simulink model "simulations"  (R2023b)
settings: Solver=VariableStepAuto  StartTime=0.0  StopTime=56  RelTol=1e-3
values from neighbouring files (symbols this model uses):
  F = pinv((Cd*(eye(4) - (Ad+Bd*K))^(-1)*Bd))    [pendulum_control.m]
  H = -KH(end)    [pendulum_control.m]
  K = - place(Ad, Bd, pK)    [pendulum_control.m]
  K_int = KH(1:end-1)    [pendulum_control.m]
  T = 0.01    [pendulum_control.m]
undefined symbols (not defined in the file or in its folder): DiscIntNeverNeededParam
libraries: cstblocks x10, eeLuenbergerObserver x5
settings Model: Creator=matia  LastModifiedBy=matia
settings SolverCC: MaxConsecutiveMinStep=3

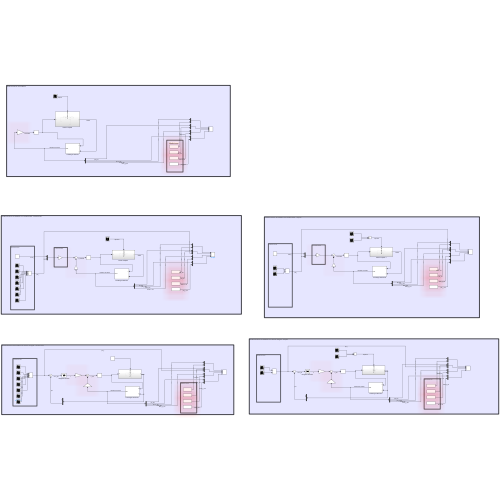
[thumbnail: Simulink's stored preview of the top-level diagram]
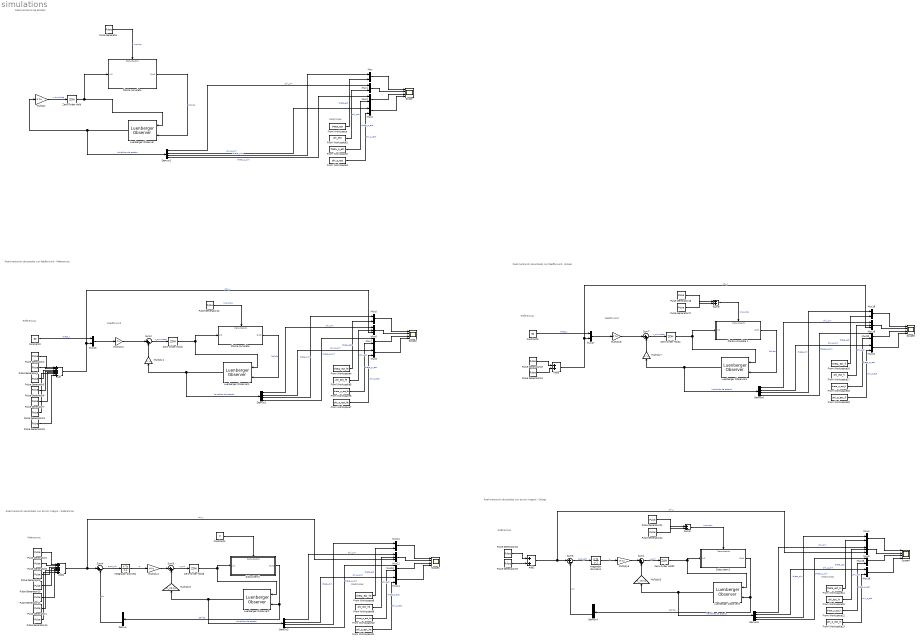
== system simulations ==
  note: Realimentación de estados con acción integral - Golpes
  note: Realimentación de estados con acción integral - Referencias
  note: Realimentación de estados con feedforward - Golpes
  note: Realimentación de estados con feedforward - Referencias
  note: Realimentación de estados
  note: Mediciones
  note: Referencias
  note: Referencias
  note: Feedforward
  note: Mediciones
  note: Referencias
  note: Mediciones
  note: Referencias
  note: Feedforward
  Add : Sum  Inputs=+++++++
  Add1 : Sum  Inputs=+++++++
  Add2 : Sum
  Add3 : Sum
  Constant1 : Constant  Value=0
  Constant2 : Constant  Value=60
  Constant3 : Constant  Value=60
  Demux : Demux  Outputs=2
  Demux{1..3,5..6} (5 alike) : Demux
  Demux4 : Demux  Outputs=2
  From Workspace : FromWorkspace  VariableName=theta_est  OutDataTypeStr=double  SampleTime=T  OutputAfterFinalValue=Setting to zero
  From Workspace1 : FromWorkspace  VariableName=phi_est  OutDataTypeStr=double  SampleTime=T  OutputAfterFinalValue=Setting to zero
  From Workspace10 : FromWorkspace  VariableName=theta_p_est_he  OutDataTypeStr=double  SampleTime=T
  From Workspace11 : FromWorkspace  VariableName=phi_p_est_he  OutDataTypeStr=double  SampleTime=T
  From Workspace12 : FromWorkspace  VariableName=theta_p_est_hi  OutDataTypeStr=double  SampleTime=T
  From Workspace13 : FromWorkspace  VariableName=phi_p_est_hi  OutDataTypeStr=double  SampleTime=T
  From Workspace14 : FromWorkspace  VariableName=theta_est_hi  OutDataTypeStr=double  SampleTime=T  OutputAfterFinalValue=Setting to zero
  From Workspace15 : FromWorkspace  VariableName=phi_est_hi  OutDataTypeStr=double  SampleTime=T
  From Workspace16 : FromWorkspace  VariableName=theta_est_fi  OutDataTypeStr=double  SampleTime=T  OutputAfterFinalValue=Setting to zero
  From Workspace17 : FromWorkspace  VariableName=phi_est_fi  SampleTime=T  OutputAfterFinalValue=Setting to zero
  From Workspace18 : FromWorkspace  VariableName=theta_p_est_fi  OutDataTypeStr=double  SampleTime=T  OutputAfterFinalValue=Setting to zero
  From Workspace19 : FromWorkspace  VariableName=phi_p_est_fi  OutDataTypeStr=double  SampleTime=T  OutputAfterFinalValue=Setting to zero
  From Workspace2 : FromWorkspace  VariableName=theta_p_est  OutDataTypeStr=double  SampleTime=T  OutputAfterFinalValue=Setting to zero
  From Workspace3 : FromWorkspace  VariableName=phi_p_est  OutDataTypeStr=double  SampleTime=T  OutputAfterFinalValue=Setting to zero
  From Workspace4 : FromWorkspace  VariableName=theta_est_fe  OutDataTypeStr=double  SampleTime=T  OutputAfterFinalValue=Setting to zero
  From Workspace5 : FromWorkspace  VariableName=phi_est_fe  OutDataTypeStr=double  SampleTime=T
  From Workspace6 : FromWorkspace  VariableName=theta_p_est_fe  OutDataTypeStr=double  SampleTime=T
  From Workspace7 : FromWorkspace  VariableName=phi_p_est_fe  OutDataTypeStr=double  SampleTime=T
  From Workspace8 : FromWorkspace  VariableName=theta_est_he  OutDataTypeStr=double  SampleTime=T  OutputAfterFinalValue=Setting to zero
  From Workspace9 : FromWorkspace  VariableName=phi_est_he  OutDataTypeStr=double  SampleTime=T
  Integrador discreto : DiscreteIntegrator  gainval=1/T  SampleTime=T  ICPrevOutput=DiscIntNeverNeededParam  ICPrevScaledInput=DiscIntNeverNeededParam
  Integrador discreto1 : DiscreteIntegrator  gainval=1/T  SampleTime=T  ICPrevOutput=DiscIntNeverNeededParam  ICPrevScaledInput=DiscIntNeverNeededParam
  Luenberger Observer{,1..4} (5 alike) : eeLuenbergerObserver/Luenberger Observer  StateSpaceType=Discrete-time  Ad=Ad  Bd=Bd  Cd=Cd  Dd=Dd  A=1  B=1  C=1  D=1  ObserverDesign=Desired eigenvalues  Ld=1  DesiredEigenvalues=pL  x0=[0;0;0;0]  Tsd=0.1  Ts=T
      settings: LibrarySourceBlock=ee_sl_lib/Observers/Luenberger Observer
  Multiply : Gain  Gain=K  Multiplication=Matrix(K*u)
  Multiply1 : Gain  Gain=K  Multiplication=Matrix(K*u)
  Multiply2 : Gain  Gain=F  Multiplication=Matrix(K*u)
  Multiply3 : Gain  Gain=K_int  Multiplication=Matrix(K*u)
  Multiply4 : Gain  Gain=H  Multiplication=Matrix(K*u)
  Multiply5 : Gain  Gain=K_int  Multiplication=Matrix(K*u)
  Multiply6 : Gain  Gain=H  Multiplication=Matrix(K*u)
  Multiply7 : Gain  Gain=K  Multiplication=Matrix(K*u)
  Multiply8 : Gain  Gain=F  Multiplication=Matrix(K*u)
  Mux{,1..5,7..8,10..11,13..18,20..21} (18 alike) : Mux  Inputs=2
  Mux{6,9,12,19} (4 alike) : Mux  Inputs=3
  Planta completa : Subsystem
      settings: PortSchema="{\"entries\":[{\"content\":{\"sides\":[{\"content\":{\"connectorIds\":[\"In1\"]},\"type\":\"ConnectorPlacement.EquallySpacedRectSide\",\"uuid\":\"327bad0f-c414-403a-b9df-5d815b8b637d\"},{\"content\":{\"connectorIds\":[\"Out1\"],\"side\":\"RIGHT\"},\"type\":\"ConnectorPlacement.EquallySpacedRectSide\",\"uuid\":\"9527d032-ecf2-4fa1-93b0-9f68fe8f2eae\"},{\"content\":{\"connectorIds\":[\"In2\"],\"side\":\"TOP\"},\"type\":\"ConnectorPlacement.EquallySpacedRectSide\",\"uuid\":\"a3d79d93-56b9-460d-b273-a140d39cea96\"}]},\"type\":\"ConnectorPlacement.EquallySpacedConnector\",\"uuid\":\"02353cda-d734-4829-adbd-41d8cd1e3a5e\"}],\"packageUris\":[\"http://schema.mathworks.com/mf0/Connector/R2020b\"],\"version\":\"1.0\"}"
  "Planta completa " : Subsystem
      settings: PortSchema="{\"entries\":[{\"content\":{\"sides\":[{\"content\":{\"connectorIds\":[\"In1\"]},\"type\":\"ConnectorPlacement.EquallySpacedRectSide\",\"uuid\":\"327bad0f-c414-403a-b9df-5d815b8b637d\"},{\"content\":{\"connectorIds\":[\"Out1\"],\"side\":\"RIGHT\"},\"type\":\"ConnectorPlacement.EquallySpacedRectSide\",\"uuid\":\"9527d032-ecf2-4fa1-93b0-9f68fe8f2eae\"},{\"content\":{\"connectorIds\":[\"In2\"],\"side\":\"TOP\"},\"type\":\"ConnectorPlacement.EquallySpacedRectSide\",\"uuid\":\"a3d79d93-56b9-460d-b273-a140d39cea96\"}]},\"type\":\"ConnectorPlacement.EquallySpacedConnector\",\"uuid\":\"02353cda-d734-4829-adbd-41d8cd1e3a5e\"}],\"packageUris\":[\"http://schema.mathworks.com/mf0/Connector/R2020b\"],\"version\":\"1.0\"}"
  Planta completa 1 : Subsystem
      settings: PortSchema="{\"entries\":[{\"content\":{\"sides\":[{\"content\":{\"connectorIds\":[\"In1\"]},\"type\":\"ConnectorPlacement.EquallySpacedRectSide\",\"uuid\":\"327bad0f-c414-403a-b9df-5d815b8b637d\"},{\"content\":{\"connectorIds\":[\"Out1\"],\"side\":\"RIGHT\"},\"type\":\"ConnectorPlacement.EquallySpacedRectSide\",\"uuid\":\"9527d032-ecf2-4fa1-93b0-9f68fe8f2eae\"},{\"content\":{\"connectorIds\":[\"In2\"],\"side\":\"TOP\"},\"type\":\"ConnectorPlacement.EquallySpacedRectSide\",\"uuid\":\"a3d79d93-56b9-460d-b273-a140d39cea96\"}]},\"type\":\"ConnectorPlacement.EquallySpacedConnector\",\"uuid\":\"02353cda-d734-4829-adbd-41d8cd1e3a5e\"}],\"packageUris\":[\"http://schema.mathworks.com/mf0/Connector/R2020b\"],\"version\":\"1.0\"}"
  Pulse Generator : DiscretePulseGenerator  PulseType=Time based  Amplitude=-8000  Period=100  PulseWidth=0.1  PhaseDelay=0.4
  Pulse Generator1 : DiscretePulseGenerator  PulseType=Time based  Amplitude=0  Period=100  PulseWidth=8  PhaseDelay=40
  Pulse Generator10 : DiscretePulseGenerator  PulseType=Time based  Amplitude=45  Period=100  PulseWidth=8  PhaseDelay=24
  Pulse Generator11 : DiscretePulseGenerator  PulseType=Time based  Amplitude=10  Period=100  PulseWidth=8  PhaseDelay=32
  Pulse Generator12 : DiscretePulseGenerator  PulseType=Time based  Amplitude=-8000  Period=100  PulseWidth=0.1  PhaseDelay=100
  Pulse Generator13 : DiscretePulseGenerator  PulseType=Time based  Amplitude=-30  Period=100  PulseWidth=8  PhaseDelay=40-0.445
  Pulse Generator14 : DiscretePulseGenerator  PulseType=Time based  Amplitude=20  Period=100  PulseWidth=8  PhaseDelay=48
  Pulse Generator15 : DiscretePulseGenerator  PulseType=Time based  Amplitude=-10  Period=100  PulseWidth=8  PhaseDelay=48-0.445
  Pulse Generator16 : DiscretePulseGenerator  PulseType=Time based  Amplitude=50000  Period=100  PulseWidth=0.01  PhaseDelay=4.77
  Pulse Generator17 : DiscretePulseGenerator  PulseType=Time based  Amplitude=-80000  Period=100  PulseWidth=0.01  PhaseDelay=25.8
  Pulse Generator18 : DiscretePulseGenerator  PulseType=Time based  Amplitude=45  Period=100  PulseWidth=20
  Pulse Generator19 : DiscretePulseGenerator  PulseType=Time based  Amplitude=-10  Period=100  PulseWidth=90  PhaseDelay=20
  Pulse Generator2 : DiscretePulseGenerator  PulseType=Time based  Amplitude=30  Period=100  PulseWidth=8
  Pulse Generator21 : DiscretePulseGenerator  PulseType=Time based  Amplitude=80000  Period=100  PulseWidth=0.01  PhaseDelay=8.136
  Pulse Generator22 : DiscretePulseGenerator  PulseType=Time based  Amplitude=80000  Period=100  PulseWidth=0.01  PhaseDelay=34.135
  Pulse Generator23 : DiscretePulseGenerator  PulseType=Time based  Amplitude=30  Period=100  PulseWidth=20
  Pulse Generator24 : DiscretePulseGenerator  PulseType=Time based  Amplitude=20  Period=100  PulseWidth=90  PhaseDelay=20
  Pulse Generator3 : DiscretePulseGenerator  PulseType=Time based  Amplitude=-20  Period=100  PulseWidth=8
  Pulse Generator4 : DiscretePulseGenerator  PulseType=Time based  Amplitude=-30  Period=100  PulseWidth=8  PhaseDelay=8-0.445
  Pulse Generator5 : DiscretePulseGenerator  PulseType=Time based  Amplitude=-10  Period=100  PulseWidth=8  PhaseDelay=16-0.445
  Pulse Generator6 : DiscretePulseGenerator  PulseType=Time based  Amplitude=20  Period=100  PulseWidth=8  PhaseDelay=24-0.445
  Pulse Generator7 : DiscretePulseGenerator  PulseType=Time based  Amplitude=0  Period=100  PulseWidth=8  PhaseDelay=32-0.445
  Pulse Generator8 : DiscretePulseGenerator  PulseType=Time based  Amplitude=0  Period=100  PulseWidth=8  PhaseDelay=8
  Pulse Generator9 : DiscretePulseGenerator  PulseType=Time based  Amplitude=20  Period=100  PulseWidth=8  PhaseDelay=16
  Scope{,2..5} (5 alike) : Scope  NumInputPorts=4
  Subsystem1 : Subsystem
      settings: PortSchema="{\"entries\":[{\"content\":{\"sides\":[{\"content\":{\"connectorIds\":[\"In1\"]},\"type\":\"ConnectorPlacement.EquallySpacedRectSide\",\"uuid\":\"327bad0f-c414-403a-b9df-5d815b8b637d\"},{\"content\":{\"connectorIds\":[\"Out1\"],\"side\":\"RIGHT\"},\"type\":\"ConnectorPlacement.EquallySpacedRectSide\",\"uuid\":\"9527d032-ecf2-4fa1-93b0-9f68fe8f2eae\"},{\"content\":{\"connectorIds\":[\"In2\"],\"side\":\"TOP\"},\"type\":\"ConnectorPlacement.EquallySpacedRectSide\",\"uuid\":\"a3d79d93-56b9-460d-b273-a140d39cea96\"}]},\"type\":\"ConnectorPlacement.EquallySpacedConnector\",\"uuid\":\"02353cda-d734-4829-adbd-41d8cd1e3a5e\"}],\"packageUris\":[\"http://schema.mathworks.com/mf0/Connector/R2020b\"],\"version\":\"1.0\"}"
  Subsystem2 : Subsystem
      settings: PortSchema="{\"entries\":[{\"content\":{\"sides\":[{\"content\":{\"connectorIds\":[\"In1\"]},\"type\":\"ConnectorPlacement.EquallySpacedRectSide\",\"uuid\":\"327bad0f-c414-403a-b9df-5d815b8b637d\"},{\"content\":{\"connectorIds\":[\"Out1\"],\"side\":\"RIGHT\"},\"type\":\"ConnectorPlacement.EquallySpacedRectSide\",\"uuid\":\"9527d032-ecf2-4fa1-93b0-9f68fe8f2eae\"},{\"content\":{\"connectorIds\":[\"In2\"],\"side\":\"TOP\"},\"type\":\"ConnectorPlacement.EquallySpacedRectSide\",\"uuid\":\"a3d79d93-56b9-460d-b273-a140d39cea96\"}]},\"type\":\"ConnectorPlacement.EquallySpacedConnector\",\"uuid\":\"02353cda-d734-4829-adbd-41d8cd1e3a5e\"}],\"packageUris\":[\"http://schema.mathworks.com/mf0/Connector/R2020b\"],\"version\":\"1.0\"}"
  Sum{1..3,6..8} (6 alike) : Sum  Inputs=|++
  Sum4 : Sum  Inputs=|+-
  Sum5 : Sum  Inputs=|+-
  Zero-Order Hold{,1..4} (5 alike) : ZeroOrderHold  SampleTime=T
  wires:
  Demux1/1 -> Mux1/1  "phi_sim"
  Demux1/3 -> Mux/1  "theta_sim"
  From Workspace/1 -> Mux/2  "theta_est"
  From Workspace1/1 -> Mux1/2  "phi_est"
  From Workspace2/1 -> Mux2/2  "theta_p_est"
  From Workspace3/1 -> Mux3/2  "phi_p_est"
  Demux1/2 -> Mux3/1  "phi_p_sim"
  Demux1/4 -> Mux2/1  "theta_p_sim"
  Mux/1 -> Scope/1
  Mux1/1 -> Scope/2
  Mux2/1 -> Scope/3
  Mux3/1 -> Scope/4
  Luenberger Observer/1 -> Multiply/1, Demux1/1  "Variables de estado"
  Demux2/3 -> Mux5/1  "theta_sim"
  Mux8/1 -> Scope2/4
  Mux5/1 -> Scope2/1
  Mux7/1 -> Scope2/3
  Mux6/1 -> Scope2/2
  Luenberger Observer1/1 -> Multiply1/1, Demux2/1  "Variables de estado"
  Demux2/1 -> Mux6/1  "phi_sim"
  Demux2/2 -> Mux8/1  "phi_p_sim"
  From Workspace6/1 -> Mux7/2  "theta_p_est"
  Demux2/4 -> Mux7/1  "theta_p_sim"
  From Workspace7/1 -> Mux8/2  "phi_p_est"
  From Workspace4/1 -> Mux5/2  "theta_est"
  "Planta completa "/1(Out1) -> Luenberger Observer1/2  "Salida"
  Multiply1/1 -> Sum2/2
  Sum2/1 -> Zero-Order Hold1/1  "u_simulada"
  Mux10/1 -> Multiply2/1
  Constant2/1 -> Mux10/1  "theta_r"
  Pulse Generator2/1 -> Add/1
  Pulse Generator4/1 -> Add/2
  Pulse Generator5/1 -> Add/3
  Pulse Generator6/1 -> Add/4
  Pulse Generator7/1 -> Add/5
  Add/1 -> Mux6/3, Mux10/2  "phi_r"
  Multiply2/1 -> Sum2/1
  Multiply4/1 -> Sum3/1
  Multiply3/1 -> Sum3/2
  Demux3/2 -> Mux14/1  "phi_p_sim"
  Luenberger Observer2/1 -> Multiply3/1, Demux3/1  "Variables de estado"
  From Workspace8/1 -> Mux11/2  "theta_est"
  Mux12/1 -> Scope3/2
  Mux13/1 -> Scope3/3
  Demux3/3 -> Mux11/1  "theta_sim"
  Subsystem2/1(Out1) -> Demux/1, Luenberger Observer2/2  "Salida"
  Mux14/1 -> Scope3/4
  Sum3/1 -> Zero-Order Hold3/1  "u_sim"
  From Workspace10/1 -> Mux13/2  "theta_p_est"
  Demux3/4 -> Mux13/1  "theta_p_sim"
  Mux11/1 -> Scope3/1
  Demux3/1 -> Mux12/1  "phi_sim"
  From Workspace11/1 -> Mux14/2  "phi_p_est"
  Sum4/1 -> Integrador discreto/1  "error_phi"
  Integrador discreto/1 -> Multiply4/1  "q"
  Pulse Generator9/1 -> Add1/3
  Pulse Generator3/1 -> Add1/1
  Pulse Generator8/1 -> Add1/2
  Pulse Generator11/1 -> Add1/5
  Pulse Generator10/1 -> Add1/4
  Add1/1 -> Mux12/3, Sum4/1  "phi_r"
  Demux/2 -> Sum4/2  "phi"
  Multiply/1 -> Zero-Order Hold/1  "u simulada"
  Pulse Generator/1 -> Planta completa/2(Perturbación)  "Impulso"
  Planta completa/1(Out1) -> Luenberger Observer/2  "Salida"
  Zero-Order Hold/1 -> Luenberger Observer/1, Planta completa/1(In2)
  Pulse Generator12/1 -> "Planta completa "/2(Perturbación)  "Impulsos"
  Constant1/1 -> Subsystem2/2(Perturbación)
  Zero-Order Hold1/1 -> "Planta completa "/1(In2), Luenberger Observer1/1
  Zero-Order Hold3/1 -> Luenberger Observer2/1, Subsystem2/1(In2)
  From Workspace9/1 -> Mux12/2  "phi_est"
  Pulse Generator1/1 -> Add1/6
  Pulse Generator14/1 -> Add1/7
  From Workspace5/1 -> Mux6/2  "phi_est"
  Pulse Generator19/1 -> Add2/2
  Mux9/1 -> Scope4/2
  Multiply6/1 -> Sum1/1
  From Workspace15/1 -> Mux9/2  "phi_est"
  Zero-Order Hold2/1 -> Luenberger Observer3/1, Subsystem1/1(In2)
  Pulse Generator18/1 -> Add2/1
  Multiply5/1 -> Sum1/2
  Mux16/1 -> Scope4/4
  Add2/1 -> Mux9/3, Sum5/1  "phi_r"
  Sum5/1 -> Integrador discreto1/1  "error_phi"
  Integrador discreto1/1 -> Multiply6/1  "q"
  Sum1/1 -> Zero-Order Hold2/1  "u_sim"
  Luenberger Observer3/1 -> Multiply5/1, Demux5/1  "Variables de estado"
  Demux5/1 -> Mux9/1  "phi_sim"
  Mux15/1 -> Scope4/3
  Demux5/4 -> Mux15/1  "theta_p_sim"
  From Workspace14/1 -> Mux4/2  "theta_est"
  Demux5/3 -> Mux4/1  "theta_sim"
  Subsystem1/1(Out1) -> Demux4/1, Luenberger Observer3/2  "Salida"
  From Workspace13/1 -> Mux16/2  "phi_p_est"
  Mux4/1 -> Scope4/1
  Demux4/2 -> Sum5/2  "phi"
  From Workspace12/1 -> Mux15/2  "theta_p_est"
  Demux5/2 -> Mux16/1  "phi_p_sim"
  Pulse Generator22/1 -> Sum6/2
  Pulse Generator21/1 -> Sum6/1
  Sum6/1 -> Subsystem1/2(Perturbación)  "Impulsos"
  Pulse Generator13/1 -> Add/6
  Pulse Generator15/1 -> Add/7
  Zero-Order Hold4/1 -> Planta completa 1/1(In2), Luenberger Observer4/1
  From Workspace17/1 -> Mux19/2  "phi_est"
  Mux20/1 -> Scope5/3
  Add3/1 -> Mux19/3, Mux17/2  "phi_r"
  Multiply8/1 -> Sum7/1
  From Workspace19/1 -> Mux21/2  "phi_p_est"
  Demux6/3 -> Mux18/1  "theta_sim"
  Mux21/1 -> Scope5/4
  Demux6/2 -> Mux21/1  "phi_p_sim"
  Demux6/1 -> Mux19/1  "phi_sim"
  Multiply7/1 -> Sum7/2
  Demux6/4 -> Mux20/1  "theta_p_sim"
  Constant3/1 -> Mux17/1  "theta_r"
  Mux18/1 -> Scope5/1
  From Workspace18/1 -> Mux20/2  "theta_p_est"
  Planta completa 1/1(Out1) -> Luenberger Observer4/2  "Salida"
  From Workspace16/1 -> Mux18/2  "theta_est"
  Pulse Generator24/1 -> Add3/2
  Pulse Generator23/1 -> Add3/1
  Mux19/1 -> Scope5/2
  Sum7/1 -> Zero-Order Hold4/1  "u_simulada"
  Mux17/1 -> Multiply8/1
  Luenberger Observer4/1 -> Multiply7/1, Demux6/1  "Variables de estado"
  Pulse Generator16/1 -> Sum8/1
  Sum8/1 -> Planta completa 1/2(Perturbación)  "Impulsos"
  Pulse Generator17/1 -> Sum8/2

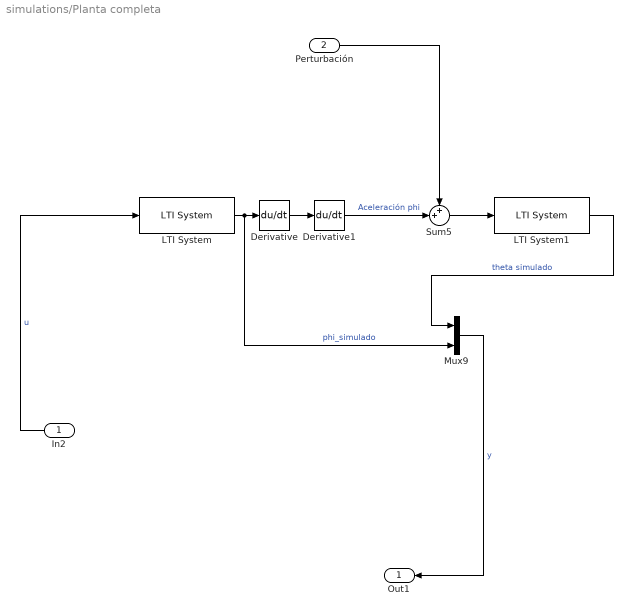
== system simulations/Planta completa ==
  In2 : Inport
  Perturbación : Inport  Port=2
  Derivative : Derivative
  Derivative1 : Derivative
  LTI System : cstblocks/LTI System  sys=Brazo  IC=[]  PadeOrder=0
  LTI System1 : cstblocks/LTI System  sys=Pe_torque  IC=[]  PadeOrder=0
  Mux9 : Mux  Inputs=2
  Sum5 : Sum  Inputs=++|  AccumDataTypeStr=single  InputSameDT=on
  Out1 : Outport
  wires:
  LTI System/1 -> Mux9/2, Derivative/1  "phi_simulado"
  Sum5/1 -> LTI System1/1
  Perturbación/1 -> Sum5/1
  Derivative1/1 -> Sum5/2  "Aceleración phi"
  LTI System1/1 -> Mux9/1  "theta simulado"
  In2/1 -> LTI System/1  "u"
  Derivative/1 -> Derivative1/1
  Mux9/1 -> Out1/1  "y"

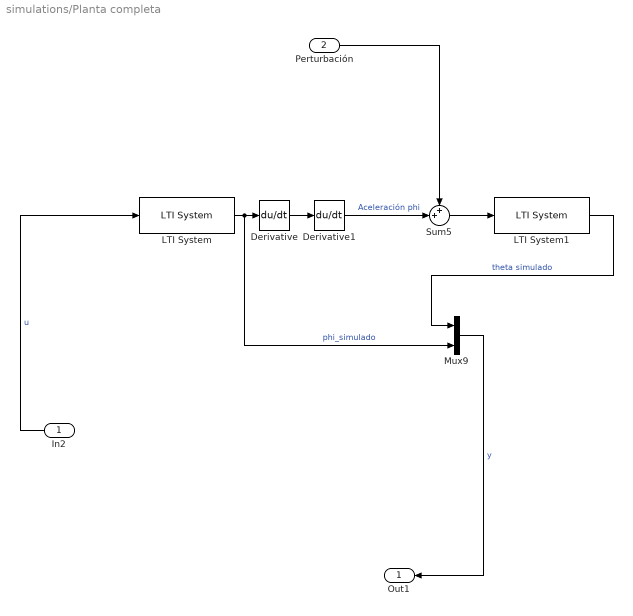
== system simulations/Planta completa  ==
  In2 : Inport
  Perturbación : Inport  Port=2
  Derivative : Derivative
  Derivative1 : Derivative
  LTI System : cstblocks/LTI System  sys=Brazo  IC=[]  PadeOrder=0
  LTI System1 : cstblocks/LTI System  sys=Pe_torque  IC=[]  PadeOrder=0
  Mux9 : Mux  Inputs=2
  Sum5 : Sum  Inputs=++|  AccumDataTypeStr=single  InputSameDT=on
  Out1 : Outport
  wires:
  LTI System/1 -> Mux9/2, Derivative/1  "phi_simulado"
  Sum5/1 -> LTI System1/1
  Perturbación/1 -> Sum5/1
  Derivative1/1 -> Sum5/2  "Aceleración phi"
  LTI System1/1 -> Mux9/1  "theta simulado"
  In2/1 -> LTI System/1  "u"
  Derivative/1 -> Derivative1/1
  Mux9/1 -> Out1/1  "y"

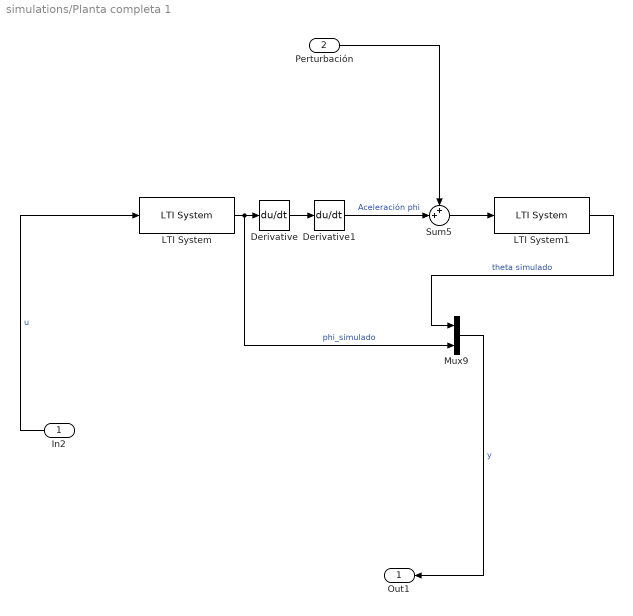
== system simulations/Planta completa 1 ==
  In2 : Inport
  Perturbación : Inport  Port=2
  Derivative : Derivative
  Derivative1 : Derivative
  LTI System : cstblocks/LTI System  sys=Brazo  IC=[]  PadeOrder=0
  LTI System1 : cstblocks/LTI System  sys=Pe_torque  IC=[]  PadeOrder=0
  Mux9 : Mux  Inputs=2
  Sum5 : Sum  Inputs=++|  AccumDataTypeStr=single  InputSameDT=on
  Out1 : Outport
  wires:
  LTI System/1 -> Mux9/2, Derivative/1  "phi_simulado"
  Sum5/1 -> LTI System1/1
  Perturbación/1 -> Sum5/1
  Derivative1/1 -> Sum5/2  "Aceleración phi"
  LTI System1/1 -> Mux9/1  "theta simulado"
  In2/1 -> LTI System/1  "u"
  Derivative/1 -> Derivative1/1
  Mux9/1 -> Out1/1  "y"

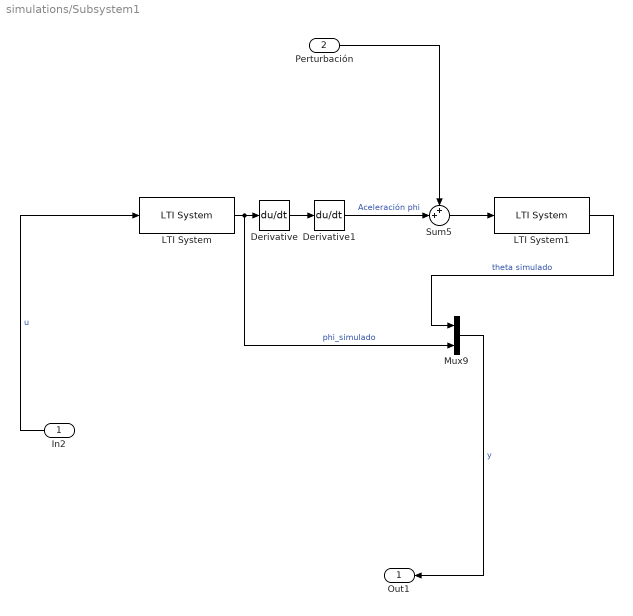
== system simulations/Subsystem1 ==
  In2 : Inport
  Perturbación : Inport  Port=2
  Derivative : Derivative
  Derivative1 : Derivative
  LTI System : cstblocks/LTI System  sys=Brazo  IC=[]  PadeOrder=0
  LTI System1 : cstblocks/LTI System  sys=Pe_torque  IC=[]  PadeOrder=0
  Mux9 : Mux  Inputs=2
  Sum5 : Sum  Inputs=++|  AccumDataTypeStr=single  InputSameDT=on
  Out1 : Outport
  wires:
  LTI System/1 -> Mux9/2, Derivative/1  "phi_simulado"
  Sum5/1 -> LTI System1/1
  Perturbación/1 -> Sum5/1
  Derivative1/1 -> Sum5/2  "Aceleración phi"
  LTI System1/1 -> Mux9/1  "theta simulado"
  In2/1 -> LTI System/1  "u"
  Derivative/1 -> Derivative1/1
  Mux9/1 -> Out1/1  "y"

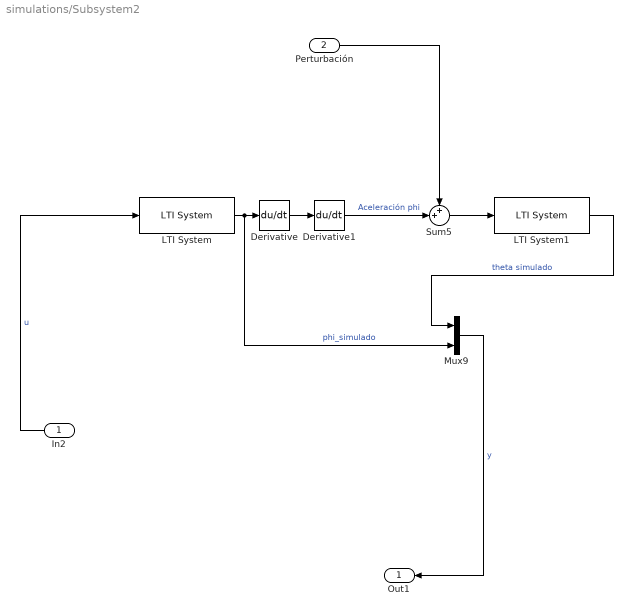
== system simulations/Subsystem2 ==
  In2 : Inport
  Perturbación : Inport  Port=2
  Derivative : Derivative
  Derivative1 : Derivative
  LTI System : cstblocks/LTI System  sys=Brazo  IC=[]  PadeOrder=0
  LTI System1 : cstblocks/LTI System  sys=Pe_torque  IC=[]  PadeOrder=0
  Mux9 : Mux  Inputs=2
  Sum5 : Sum  Inputs=++|  AccumDataTypeStr=single  InputSameDT=on
  Out1 : Outport
  wires:
  LTI System/1 -> Mux9/2, Derivative/1  "phi_simulado"
  Sum5/1 -> LTI System1/1
  Perturbación/1 -> Sum5/1
  Derivative1/1 -> Sum5/2  "Aceleración phi"
  LTI System1/1 -> Mux9/1  "theta simulado"
  In2/1 -> LTI System/1  "u"
  Derivative/1 -> Derivative1/1
  Mux9/1 -> Out1/1  "y"
